simulink library "monroe_library"  (R2012b)
settings: Solver=ode45  StartTime=0.0  StopTime=10.0  RelTol=1e-3
values from neighbouring files (symbols this model uses):
  input_bit_width = ', num2str(input_bit_width))    [fft_direct_draw.m]
undefined symbols (not defined in the file or in its folder): gcbh, xlBlockLoadCallback
libraries: xbsIndex_r4 x1880, monroe_library x159, casper_library x13, xps_library x1
(part 2 of 43)

== system monroe_library/coeff_gen_dual ==
  sync : Inport
  Concat : xbsIndex_r4/Concat  num_inputs=2  dbl_ovrd=off  block_type=concat
  Concat1 : xbsIndex_r4/Concat  num_inputs=2  dbl_ovrd=off  block_type=concat
  Concat2 : xbsIndex_r4/Concat  num_inputs=2  dbl_ovrd=off  block_type=concat
  Constant : xbsIndex_r4/Constant  arith_type=Boolean  const=0  n_bits=16  bin_pt=14  explicit_period=on  period=1  equ=P=C  opselect=C  inp2=PCIN>>17  opr=+  inp1=P  carry=CIN  dbl_ovrd=off  block_type=constant
  Constant1 : xbsIndex_r4/Constant  arith_type=Boolean  const=1  n_bits=16  bin_pt=14  explicit_period=off  period=1  equ=P=C  opselect=C  inp2=PCIN>>17  opr=+  inp1=P  carry=CIN  dbl_ovrd=off  block_type=constant
  Constant3 : xbsIndex_r4/Constant  arith_type=Signed (2's comp)  const=0  n_bits=18  bin_pt=17  explicit_period=on  period=1  equ=P=C  opselect=C  inp2=PCIN>>17  opr=+  inp1=P  carry=CIN  dbl_ovrd=off  block_type=constant
  Constant4 : xbsIndex_r4/Constant  arith_type=Boolean  const=0  n_bits=16  bin_pt=14  explicit_period=off  period=1  equ=P=C  opselect=C  inp2=PCIN>>17  opr=+  inp1=P  carry=CIN  dbl_ovrd=off  block_type=constant
  Constant5 : xbsIndex_r4/Constant  arith_type=Unsigned  const=2  n_bits=6  bin_pt=0  explicit_period=on  period=1  equ=P=C  opselect=C  inp2=PCIN>>17  opr=+  inp1=P  carry=CIN  dbl_ovrd=off  block_type=constant
  Counter : xbsIndex_r4/Counter  cnt_type=Free Running  cnt_to=Inf  operation=Up  start_count=0  cnt_by_val=1  arith_type=Unsigned  n_bits=6  bin_pt=0  load_pin=on  rst=off  en=off  explicit_period=on  period=1  dbl_ovrd=off  use_behavioral_HDL=off  implementation=Fabric  block_type=counter
  Delay : xbsIndex_r4/Delay  en=off  latency=0  dbl_ovrd=off  reg_retiming=off  block_type=delay
  Dual Port RAM4 : xbsIndex_r4/Dual Port RAM  depth=128  initVector=[0.0078125 0.015625 0.0234375 0.03125 0.0390625 0.046875 0.0546875 0.0625 0.0703125 0.078125 0.0859375 0.09375 0.1015625 0.109375 0.1171875 0.125 0.1328125 0.140625 0.1484375 0.15625 0.1640625 0.171875 0.1796875 0.1875 0.1953125 0.203125 0.2109375 0.21875 0.2265625 0.234375 0.2421875 0.25 0.2578125 0.265625 0.2734375 0.28125 0.2890625 0.296875 0.3046875 0.3125 0.3203125 0.328125 0.3359375 0.34375 0.3515625 0.359375 0.3671875 0.375 0.3828125 0.390625 0.3984375 0.40625 0.4140625 0.421875 0.4296875 0.4375 0.4453125 0.453125 0.4609375 0.46875 0.4765625 0.484375 0.4921875 0.5 0.5078125 0.515625 0.5234375 0.53125 0.5390625 0.546875 0.5546875 0.5625 0.5703125 0.578125 0.5859375 0.59375 0.6015625 0.609375 0.6171875 0.625 0.6328125 0.640625 0.6484375 0.65625 0.6640625 0.671875 0.6796875 0.6875 0.6953125 0.703125 0.7109375 0.71875 0.7265625 0.734375 0.7421875 0.75 0.7578125 0.765625 0.7734375 0.78125 0.7890625 0.796875 0.8046875 0.8125 0.8203125 0.828125 0.8359375 0.84375 0.8515625 0.859375 0.8671875 0.875 0.8828125 0.890625 0.8984375 0.90625 0.9140625 0.921875 0.9296875 0.9375 0.9453125 0.953125 0.9609375 0.96875 0.9765625 0.984375 0.9921875 1]  distributed_mem=Block RAM  init_a=0  init_b=0  rst_a=off  rst_b=off  en_a=off  en_b=off  latency=2  write_mode_A=No Read On Write  write_mode_B=No Read On Write  dbl_ovrd=off  optimize=Area  use_rpm=on  block_type=dpram
  Reinterpret : xbsIndex_r4/Reinterpret  force_arith_type=on  arith_type=Unsigned  force_bin_pt=on  bin_pt=0  block_type=reinterpret
      settings: infoedit="Changes signal type without altering the binary representation.   You can changed the signal between signed and unsigned, and relocate the binary point.<br><br>Hardware notes: In hardware this block costs nothing.<br><br>Example:  Suppose the input is 6 bits wide, signed, with 2 fractional bits, and the output is forced to unsigned with 0 fractional bits.  Then an input of -2.0 (1110.00 in binary 2's complement) becomes an output of 56 (111000 in binary)."
  Reinterpret1 : xbsIndex_r4/Reinterpret  force_arith_type=on  arith_type=Unsigned  force_bin_pt=on  bin_pt=0  block_type=reinterpret
      settings: infoedit="Changes signal type without altering the binary representation.   You can changed the signal between signed and unsigned, and relocate the binary point.<br><br>Hardware notes: In hardware this block costs nothing.<br><br>Example:  Suppose the input is 6 bits wide, signed, with 2 fractional bits, and the output is forced to unsigned with 0 fractional bits.  Then an input of -2.0 (1110.00 in binary 2's complement) becomes an output of 56 (111000 in binary)."
  count_slice : xbsIndex_r4/Slice  nbits=6  boolean_output=off  mode=Upper Bit Location + Width  bit1=0  base1=MSB of Input  bit0=0  base0=MSB of Input  dbl_ovrd=off  block_type=slice
  coeff : Outport
  wires:
  count_slice/1 -> Concat1/2, Concat/2  "xlsub2_Counter_out1"
  Constant3/1 -> Dual Port RAM4/5, Dual Port RAM4/2  "xlsub2_Constant3_out1"
  Constant/1 -> Dual Port RAM4/6, Dual Port RAM4/3  "xlsub2_Constant_out1"
  Reinterpret1/1 -> Concat2/2  "xlsub2_Reinterpret1_out1"
  Dual Port RAM4/2 -> Reinterpret1/1  "xlsub2_Dual_Port_RAM4_out2"
  Reinterpret/1 -> Concat2/1  "xlsub2_Reinterpret_out1"
  Dual Port RAM4/1 -> Reinterpret/1  "xlsub2_Dual_Port_RAM4_out1"
  Concat1/1 -> Dual Port RAM4/4  "xlsub2_Concat1_out1"
  Concat/1 -> Dual Port RAM4/1  "xlsub2_Concat_out1"
  Delay/1 -> coeff/1
  Concat2/1 -> Delay/1  "xlsub2_Concat2_out1"
  Counter/1 -> count_slice/1
  Constant5/1 -> Counter/2  "xlsub2_Constant5_out1"
  sync/1 -> Counter/1
  Constant4/1 -> Concat1/1  "xlsub2_Constant4_out1"
  Constant1/1 -> Concat/1  "xlsub2_Constant1_out1"

== system monroe_library/counter_limited_fast ==
  Constant : xbsIndex_r4/Constant  arith_type=Unsigned  const=count_to - 2  n_bits=bit_width  bin_pt=0  explicit_period=off  period=1  equ=P=C  opselect=C  inp2=PCIN>>17  opr=+  inp1=P  carry=CIN  dbl_ovrd=off  block_type=constant
      settings: block_version=11.4
  Constant1 : xbsIndex_r4/Constant  arith_type=Boolean  const=cheap_counter  n_bits=16  bin_pt=14  explicit_period=off  period=1  equ=P=C  opselect=C  inp2=PCIN>>17  opr=+  inp1=P  carry=CIN  dbl_ovrd=off  block_type=constant
  Counter : xbsIndex_r4/Counter  cnt_type=Free Running  cnt_to=250  operation=Up  start_count=0  cnt_by_val=1  arith_type=Unsigned  n_bits=bit_width  bin_pt=0  load_pin=off  rst=on  en=off  explicit_period=on  period=1  dbl_ovrd=off  use_behavioral_HDL=off  implementation=Fabric  use_rpm=off  block_type=counter
      settings: xl_area=[0, 0, 0, 0, 0, 0, 0]  block_version=9.1.01
  Counter1 : S-Function  LoadFcn=xlBlockLoadCallback(gcbh);  FunctionName=sysgen  Parameters=ptable_  EnableBusSupport=off  mask(Xilinx Counter Block){infoedit=Hardware notes: Free running counters are the least expensive in hardware.  A count limited counter is implemented by combining a counter with a comparator., cnt_type_sgadvanced=, cnt_type=Count Limited, cnt_to=count_to, operation_sgadvanced=, operation=Up, start_count=0, cnt_by_val=1, arith_type_sgadvanced=, arith_type=Unsigned, n_bits=bit_width, bin_pt=0, load_pin_sgadvanced=, load_pin=off, rst_sgadvanced=, rst=off, en_sgadvanced=, en=off, explicit_period_sgadvanced=, explicit_period=on, period=1, dbl_ovrd_sgadvanced=, dbl_ovrd=off, use_behavioral_HDL_sgadvanced=, use_behavioral_HDL=off, implementation_sgadvanced=, implementation=Fabric, xl_use_area_sgadvanced=, xl_use_area=off, xl_area=[0, 0, 0, 0, 0, 0, 0], use_rpm=off, xlcconfig=, has_advanced_control=0, sggui_pos=862,137,419,748, block_type=counter, block_version=9.1.01, sg_icon_stat=40,40,0,1,white,blue,0,4b061529,right,,[ ],[ ], sg_mask_display=|, sg_list_contents=, sg_blockgui_xml=}
      mask sg_mask_display=|
      | fprintf('','COMMENT: begin icon graphics');
      | patch([0 40 40 0 0 ],[0 0 40 40 0 ],[0.77 0.82 0.91 ]);
      | plot([0 40 40 0 0 ],[0 0 40 40 0 ]);
      | patch([8.875 16.1 21.1 26.1 31.1 21.1 13.875 8.875 ],[25.55 25.55 30.55 25.55 30.55 30.55 30.55 25.55 ],[1 1 1 ]);
      | patch([13.875 21.1 16.1 8.875 13.875 ],[20.55 20.55 25.55 25.55 20.55 ],[0.931 0.946 0.973 ]);
      | patch([8.875 16.1 21.1 13.875 8.875 ],[15.55 15.55 20.55 20.55 15.55 ],[1 1 1 ]);
      | patch([13.875 31.1 26.1 21.1 16.1 8.875 13.875 ],[10.55 10.55 15.55 10.55 15.55 15.55 10.55 ],[0.931 0.946 0.973 ]);
      | fprintf('','COMMENT: end icon graphics');
      | fprintf('','COMMENT: begin icon text');
      |
      | color('black');disp('{\fontsize{14}\bf\lceil++\rceil}','texmode','on');
      | fprintf('','COMMENT: end icon text');
      mask prompts: infoedit ""; cnt_type_sgadvanced ""; cnt_type "Counter type"; cnt_to "Count to value"; operation_sgadvanced ""; operation "Count direction"; start_count "Initial value"; cnt_by_val "Step"; arith_type_sgadvanced ""; arith_type "Output type"; n_bits "Number of bits"; bin_pt "Binary point"; load_pin_sgadvanced ""; load_pin "Provide load port"; rst_sgadvanced ""; rst "Provide synchronous reset port"; en_sgadvanced ""; en "Provide enable port"; explicit_period_sgadvanced ""; explicit_period "Sample period source"; period "Explicit period"; dbl_ovrd_sgadvanced ""; dbl_ovrd "Override with doubles"; use_behavioral_HDL_sgadvanced ""; use_behavioral_HDL "Use behavioral HDL (otherwise use core)"; implementation_sgadvanced ""; implementation "Implement using"; xl_use_area_sgadvanced ""; xl_use_area "Define FPGA area for resource estimation"; xl_area "FPGA area [slices, FFs, BRAMs, LUTs, IOBs, emb. mults, TBUFs]"; use_rpm ""; xlcconfig ""; has_advanced_control ""; sggui_pos ""; block_type ""; block_version ""; sg_icon_stat ""; sg_mask_display ""; sg_list_contents ""; sg_blockgui_xml ""
      mask help: Hardware notes: Free running counters are the least expensive in hardware. A count limited counter is implemented by combining a counter with a comparator.
      mask init:
      | try
      |   tmp_gcb = gcb;
      |   tmp_gcbh = gcbh;
      |   if (strcmp('SysGenIndex',get_param(bdroot(tmp_gcbh),'tag')) && ~isempty(regexp(bdroot(tmp_gcb), '^xbs', 'once')))
      |     return;
      |   end;
      |   xlMungeMaskParams;
      |   block_config = 'sysgen_blockset:Counter_config';
      | 
      |   block_type='counter';
      | 
      |   serialized_declarations = '{''arith_type''=>''Int'',''bin_pt''=>''Int'',''cnt_by_val''=>''Double'',''cnt_to''=>''Double'',''cnt_type''=>''Int'',''en''=>''Int'',''explicit_period''=>''Int'',''implementation''=>''String'',''load_pin''=>''Int'',''n_bits''=>''Int'',''operation''=>''Int'',''period''=>''Double'',''rst''=>''Int'',''start_count''=>''Double'',''use_behavioral_HDL''=>''Int'',''use_rpm''=>''String'',''xlcconfig''=>''String'',''block_type''=>''String''}';
      |   ptable_ = xlblockprep(get_param(tmp_gcb, 'MaskWSVariables'));
      |   try
      |     xlBlockMoveCallback(tmp_gcbh);
      |   catch 
      |      clear global xl_updateicon_recursion_guard;
      |   end;
      | catch
      |   global dbgsysgen;
      |   if(~isempty(dbgsysgen) && dbgsysgen)
      |     e = regexprep(lasterr, '\n', '\nError: ');
      |     disp(['Error: While running MaskInit code on block ' tmp_gcb ': ' e]);
      |     error(e);
      |   end
      | end
      settings: CopyFcn=xlBlockMoveCallback(gcbh);  DeleteFcn=xlDestroyGui(gcbh);  ModelCloseFcn=xlDestroyGui(gcbh);  PreSaveFcn=xlBlockPreSaveCallback(gcbh);  PostSaveFcn=xlBlockPostSaveCallback(gcbh);  DestroyFcn=xlDestroyGui(gcbh);  OpenFcn=xlOpenGui(gcbh, 'counter_gui.xml', @counterenablement, -1)  CloseFcn=xlDestroyGui(gcbh);  MoveFcn=xlBlockMoveCallback(gcbh);
      mask Help: eval('');xlDoc('-book','sysgen','-topic','Counter');
      mask TypeOptions cnt_type: Free Running | Count Limited
      mask TypeOptions operation: Up | Down | Up/Down
      mask TypeOptions arith_type: Signed  (2's comp) | Unsigned
      mask TypeOptions explicit_period: on | off
      mask TypeOptions implementation: Fabric | DSP48
      mask Display:
      | fprintf('','COMMENT: begin icon graphics');
      | patch([0 40 40 0 0 ],[0 0 40 40 0 ],[0.77 0.82 0.91 ]);
      | plot([0 40 40 0 0 ],[0 0 40 40 0 ]);
      | patch([8.875 16.1 21.1 26.1 31.1 21.1 13.875 8.875 ],[25.55 25.55 30.55 25.55 30.55 30.55 30.55 25.55 ],[1 1 1 ]);
      | patch([13.875 21.1 16.1 8.875 13.875 ],[20.55 20.55 25.55 25.55 20.55 ],[0.931 0.946 0.973 ]);
      | patch([8.875 16.1 21.1 13.875 8.875 ],[15.55 15.55 20.55 20.55 15.55 ],[1 1 1 ]);
      | patch([13.875 31.1 26.1 21.1 16.1 8.875 13.875 ],[10.55 10.55 15.55 10.55 15.55 15.55 10.55 ],[0.931 0.946 0.973 ]);
      | fprintf('','COMMENT: end icon graphics');
      | fprintf('','COMMENT: begin icon text');
      | 
      | color('black');disp('{\fontsize{14}\bf\lceil++\rceil}','texmode','on');
      | fprintf('','COMMENT: end icon text');
  Delay : xbsIndex_r4/Delay  en=off  latency=1  dbl_ovrd=off  reg_retiming=off  block_type=delay
      settings: block_version=11.4
  Delay1 : S-Function  LoadFcn=xlBlockLoadCallback(gcbh);  FunctionName=sysgen  Parameters=ptable_  EnableBusSupport=off  mask(Xilinx Delay Block){infoedit=Hardware notes: A delay line is a chain, each link of which is an SRL16 followed by a flip-flop., en_sgadvanced=, en=off, latency=register_output, dbl_ovrd_sgadvanced=, dbl_ovrd=off, reg_retiming_sgadvanced=, reg_retiming=off, xl_use_area_sgadvanced=, xl_use_area=off, xl_area=[0,0,0,0,0,0,0], has_advanced_control=0, sggui_pos=-1,-1,-1,-1, block_type=delay, block_version=11.4, sg_icon_stat=60,56,1,1,white,blue,0,24450e6f,right,,[ ],[ ], sg_mask_display=|, sg_list_contents=, sg_blockgui_xml=}
      mask sg_mask_display=|
      | fprintf('','COMMENT: begin icon graphics');
      | patch([0 60 60 0 0 ],[0 0 56 56 0 ],[0.77 0.82 0.91 ]);
      | plot([0 60 60 0 0 ],[0 0 56 56 0 ]);
      | patch([12.2 23.76 31.76 39.76 47.76 31.76 20.2 12.2 ],[36.88 36.88 44.88 36.88 44.88 44.88 44.88 36.88 ],[1 1 1 ]);
      | patch([20.2 31.76 23.76 12.2 20.2 ],[28.88 28.88 36.88 36.88 28.88 ],[0.931 0.946 0.973 ]);
      | patch([12.2 23.76 31.76 20.2 12.2 ],[20.88 20.88 28.88 28.88 20.88 ],[1 1 1 ]);
      | patch([20.2 47.76 39.76 31.76 23.76 12.2 20.2 ],[12.88 12.88 20.88 12.88 20.88 20.88 12.88 ],[0.931 0.946 0.973 ]);
      | fprintf('','COMMENT: end icon graphics');
      | fprintf('','COMMENT: begin icon text');
      |
      |
      | color('black');disp('z^{-0}','texmode','on');
      | fprintf('','COMMENT: end icon text');
      mask prompts: infoedit ""; en_sgadvanced ""; en "Provide enable port"; dbl_ovrd_sgadvanced ""; dbl_ovrd "Override with doubles"; reg_retiming_sgadvanced ""; reg_retiming "Implement using behavioral HDL."; xl_use_area_sgadvanced ""; xl_use_area "Define FPGA area for resource estimation"; xl_area "FPGA area [slices, FFs, BRAMs, LUTs, IOBs, emb. mults, TBUFs]"; has_advanced_control ""; sggui_pos ""; block_type ""; block_version ""; sg_icon_stat ""; sg_mask_display ""; sg_list_contents ""; sg_blockgui_xml ""
      mask help: Hardware notes: A delay line is a chain, each link of which is an SRL16 followed by a flip-flop.
      mask init:
      | try
      |   tmp_gcb = gcb;
      |   tmp_gcbh = gcbh;
      |   if (strcmp('SysGenIndex',get_param(bdroot(tmp_gcbh),'tag')) && ~isempty(regexp(bdroot(tmp_gcb), '^xbs', 'once')))
      |     return;
      |   end;
      |   xlMungeMaskParams;
      |   block_config = 'sysgen_blockset:Delay_config';
      | 
      |   block_type='delay';
      | 
      |   serialized_declarations = '{''dbl_ovrd''=>''Int'',''en''=>''Int'',''latency''=>''Int'',''reg_retiming''=>''Int'',''block_type''=>''String''}';
      |   ptable_ = xlblockprep(get_param(tmp_gcb, 'MaskWSVariables'));
      |   try
      |     xlBlockMoveCallback(tmp_gcbh);
      |   catch 
      |      clear global xl_updateicon_recursion_guard;
      |   end;
      | catch
      |   global dbgsysgen;
      |   if(~isempty(dbgsysgen) && dbgsysgen)
      |     e = regexprep(lasterr, '\n', '\nError: ');
      |     disp(['Error: While running MaskInit code on block ' tmp_gcb ': ' e]);
      |     error(e);
      |   end
      | end
      settings: CopyFcn=xlBlockMoveCallback(gcbh);  DeleteFcn=xlDestroyGui(gcbh);  ModelCloseFcn=xlDestroyGui(gcbh);  PreSaveFcn=xlBlockPreSaveCallback(gcbh);  PostSaveFcn=xlBlockPostSaveCallback(gcbh);  DestroyFcn=xlDestroyGui(gcbh);  OpenFcn=xlOpenGui(gcbh, 'delay_gui.xml', @xlmagicenablement, -1)  CloseFcn=xlDestroyGui(gcbh);  MoveFcn=xlBlockMoveCallback(gcbh);
      mask Help: eval('');xlDoc('-book','sysgen','-topic','Delay');
      mask Display:
      | fprintf('','COMMENT: begin icon graphics');
      | patch([0 60 60 0 0 ],[0 0 56 56 0 ],[0.77 0.82 0.91 ]);
      | plot([0 60 60 0 0 ],[0 0 56 56 0 ]);
      | patch([12.2 23.76 31.76 39.76 47.76 31.76 20.2 12.2 ],[36.88 36.88 44.88 36.88 44.88 44.88 44.88 36.88 ],[1 1 1 ]);
      | patch([20.2 31.76 23.76 12.2 20.2 ],[28.88 28.88 36.88 36.88 28.88 ],[0.931 0.946 0.973 ]);
      | patch([12.2 23.76 31.76 20.2 12.2 ],[20.88 20.88 28.88 28.88 20.88 ],[1 1 1 ]);
      | patch([20.2 47.76 39.76 31.76 23.76 12.2 20.2 ],[12.88 12.88 20.88 12.88 20.88 20.88 12.88 ],[0.931 0.946 0.973 ]);
      | fprintf('','COMMENT: end icon graphics');
      | fprintf('','COMMENT: begin icon text');
      | 
      | 
      | color('black');disp('z^{-0}','texmode','on');
      | fprintf('','COMMENT: end icon text');
  Delay2 : monroe_library/counter_limited_fast/Delay1  en=off  latency=1  dbl_ovrd=off  reg_retiming=off  block_type=delay
      settings: infoedit=Hardware notes: A delay line is a chain, each link of which is an SRL16 followed by a flip-flop.  block_version=11.4
  Delay3 : S-Function  LoadFcn=xlBlockLoadCallback(gcbh);  FunctionName=sysgen  Parameters=ptable_  EnableBusSupport=off  mask(Xilinx Delay Block){infoedit=Hardware notes: A delay line is a chain, each link of which is an SRL16 followed by a flip-flop., en_sgadvanced=, en=off, latency=register_output, dbl_ovrd_sgadvanced=, dbl_ovrd=off, reg_retiming_sgadvanced=, reg_retiming=off, xl_use_area_sgadvanced=, xl_use_area=off, xl_area=[0,0,0,0,0,0,0], has_advanced_control=0, sggui_pos=-1,-1,-1,-1, block_type=delay, block_version=11.4, sg_icon_stat=60,56,1,1,white,blue,0,24450e6f,right,,[ ],[ ], sg_mask_display=|, sg_list_contents=, sg_blockgui_xml=}
      mask sg_mask_display=|
      | fprintf('','COMMENT: begin icon graphics');
      | patch([0 60 60 0 0 ],[0 0 56 56 0 ],[0.77 0.82 0.91 ]);
      | plot([0 60 60 0 0 ],[0 0 56 56 0 ]);
      | patch([12.2 23.76 31.76 39.76 47.76 31.76 20.2 12.2 ],[36.88 36.88 44.88 36.88 44.88 44.88 44.88 36.88 ],[1 1 1 ]);
      | patch([20.2 31.76 23.76 12.2 20.2 ],[28.88 28.88 36.88 36.88 28.88 ],[0.931 0.946 0.973 ]);
      | patch([12.2 23.76 31.76 20.2 12.2 ],[20.88 20.88 28.88 28.88 20.88 ],[1 1 1 ]);
      | patch([20.2 47.76 39.76 31.76 23.76 12.2 20.2 ],[12.88 12.88 20.88 12.88 20.88 20.88 12.88 ],[0.931 0.946 0.973 ]);
      | fprintf('','COMMENT: end icon graphics');
      | fprintf('','COMMENT: begin icon text');
      |
      |
      | color('black');disp('z^{-0}','texmode','on');
      | fprintf('','COMMENT: end icon text');
      mask prompts: infoedit ""; en_sgadvanced ""; en "Provide enable port"; dbl_ovrd_sgadvanced ""; dbl_ovrd "Override with doubles"; reg_retiming_sgadvanced ""; reg_retiming "Implement using behavioral HDL."; xl_use_area_sgadvanced ""; xl_use_area "Define FPGA area for resource estimation"; xl_area "FPGA area [slices, FFs, BRAMs, LUTs, IOBs, emb. mults, TBUFs]"; has_advanced_control ""; sggui_pos ""; block_type ""; block_version ""; sg_icon_stat ""; sg_mask_display ""; sg_list_contents ""; sg_blockgui_xml ""
      mask help: Hardware notes: A delay line is a chain, each link of which is an SRL16 followed by a flip-flop.
      mask init: same as monroe_library/counter_limited_fast/Delay1
      settings: CopyFcn=xlBlockMoveCallback(gcbh);  DeleteFcn=xlDestroyGui(gcbh);  ModelCloseFcn=xlDestroyGui(gcbh);  PreSaveFcn=xlBlockPreSaveCallback(gcbh);  PostSaveFcn=xlBlockPostSaveCallback(gcbh);  DestroyFcn=xlDestroyGui(gcbh);  OpenFcn=xlOpenGui(gcbh, 'delay_gui.xml', @xlmagicenablement, -1)  CloseFcn=xlDestroyGui(gcbh);  MoveFcn=xlBlockMoveCallback(gcbh);
      mask Help: eval('');xlDoc('-book','sysgen','-topic','Delay');
      mask Display:
      | fprintf('','COMMENT: begin icon graphics');
      | patch([0 60 60 0 0 ],[0 0 56 56 0 ],[0.77 0.82 0.91 ]);
      | plot([0 60 60 0 0 ],[0 0 56 56 0 ]);
      | patch([12.2 23.76 31.76 39.76 47.76 31.76 20.2 12.2 ],[36.88 36.88 44.88 36.88 44.88 44.88 44.88 36.88 ],[1 1 1 ]);
      | patch([20.2 31.76 23.76 12.2 20.2 ],[28.88 28.88 36.88 36.88 28.88 ],[0.931 0.946 0.973 ]);
      | patch([12.2 23.76 31.76 20.2 12.2 ],[20.88 20.88 28.88 28.88 20.88 ],[1 1 1 ]);
      | patch([20.2 47.76 39.76 31.76 23.76 12.2 20.2 ],[12.88 12.88 20.88 12.88 20.88 20.88 12.88 ],[0.931 0.946 0.973 ]);
      | fprintf('','COMMENT: end icon graphics');
      | fprintf('','COMMENT: begin icon text');
      | 
      | 
      | color('black');disp('z^{-0}','texmode','on');
      | fprintf('','COMMENT: end icon text');
  Mux : xbsIndex_r4/Mux  inputs=2  en=off  latency=0  precision=Full  arith_type=Unsigned  n_bits=16  bin_pt=14  quantization=Truncate  overflow=Wrap  dbl_ovrd=off  block_type=mux
  Relational : xbsIndex_r4/Relational  mode=a=b  en=off  latency=0  dbl_ovrd=off  block_type=relational
  count : Outport
  wires:
  Delay/1 -> Relational/2, Delay1/1
  Constant/1 -> Relational/1
  Counter/1 -> Delay/1
  Relational/1 -> Delay2/1
  Delay2/1 -> Counter/1
  Counter1/1 -> Delay3/1
  Delay3/1 -> Mux/3
  Delay1/1 -> Mux/2
  Constant1/1 -> Mux/1
  Mux/1 -> count/1

== system monroe_library/cram ==
  in0 : Inport
  in1 : Inport  Port=2
  in2 : Inport  Port=3
  in3 : Inport  Port=4
  in4 : Inport  Port=5
  in5 : Inport  Port=6
  concat : xbsIndex_r4/Concat  num_inputs=6  dbl_ovrd=off  block_type=concat
  reinterpret_{1..6} (6 alike) : xbsIndex_r4/Reinterpret  force_arith_type=on  arith_type=Unsigned  force_bin_pt=on  bin_pt=0  block_type=reinterpret
      settings: infoedit="Changes signal type without altering the binary representation.   You can changed the signal between signed and unsigned, and relocate the binary point.<br><br>Hardware notes: In hardware this block costs nothing.<br><br>Example:  Suppose the input is 6 bits wide, signed, with 2 fractional bits, and the output is forced to unsigned with 0 fractional bits.  Then an input of -2.0 (1110.00 in binary 2's complement) becomes an output of 56 (111000 in binary)."
  out : Outport
  wires:
  concat/1 -> out/1
  reinterpret_6/1 -> concat/6
  reinterpret_5/1 -> concat/5
  reinterpret_4/1 -> concat/4
  reinterpret_3/1 -> concat/3
  reinterpret_2/1 -> concat/2
  reinterpret_1/1 -> concat/1
  in5/1 -> reinterpret_6/1
  in4/1 -> reinterpret_5/1
  in3/1 -> reinterpret_4/1
  in2/1 -> reinterpret_3/1
  in1/1 -> reinterpret_2/1
  in0/1 -> reinterpret_1/1

== system monroe_library/delay_bram_fast ==
  in : Inport
  Constant2 : xbsIndex_r4/Constant  arith_type=Boolean  const=1  n_bits=1  bin_pt=0  explicit_period=on  period=1  equ=P=C  opselect=C  inp2=PCIN>>17  opr=+  inp1=P  carry=CIN  dbl_ovrd=off  block_type=constant
      settings: block_version=9.1.01
  Single Port RAM : xbsIndex_r4/Single Port RAM  depth=delay_len-bram_latency  initVector=0  distributed_mem=Block RAM  write_mode=Read Before Write  rst=off  init_reg=0  en=off  latency=bram_latency  dbl_ovrd=off  optimize=Area  use_rpm=off  block_type=spram
      settings: xl_area=[0, 0, 0, 0, 0, 0, 0]  block_version=9.1.01
  counter_limited_fast : monroe_library/counter_limited_fast  SystemSampleTime=-1  bit_width=ceil(log(delay_len-bram_latency)/log(2))  count_to=delay_len-bram_latency-1  register_output=register_counter  cheap_counter=((ceil(log(delay_len-bram_latency)/log(2))) < 8)
  out : Outport
  wires:
  counter_limited_fast/1 -> Single Port RAM/1
  Constant2/1 -> Single Port RAM/3
  in/1 -> Single Port RAM/2
  Single Port RAM/1 -> out/1
